simulink model "Galvo_sys_v14"  (R2013a)
settings: Solver=ode45  StartTime=0.0  StopTime=10e-3  MaxStep=1e-4  RelTol=1e-3
InitFcn:
  | Kp_cc = evalin('base','Kp_cc');
StartFcn:
  | Kp_cc = evalin('base','Kp_cc')
model workspace (MATLAB code in the model file):
  | Kp_cc = evalin('base','Kp_cc');
libraries: simulink x2
settings Model: Kp_cc=1  Creator=mainster  LastModifiedBy=mainster
settings DataIOCC: SaveFormat=StructureWithTime

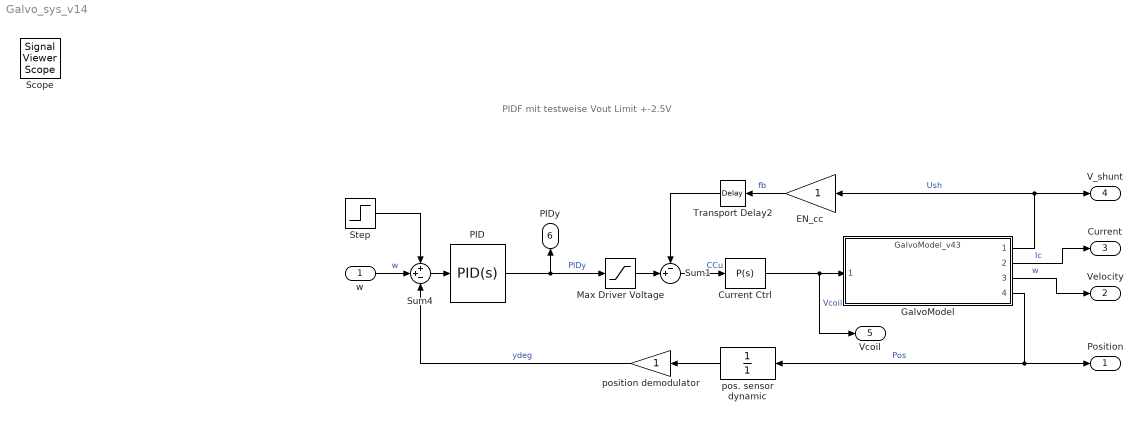
== system Galvo_sys_v14 ==
  note: PIDF mit testweise Vout Limit +-2.5V
  w : Inport
  Current Ctrl : simulink/Continuous/PID Controller  Controller=P  TimeDomain=Continuous-time  SampleTime=1  IntegratorMethod=Forward Euler  FilterMethod=Forward Euler  Form=Parallel  P=Kp_cc  I=1  D=0  N=100  InitialConditionSource=internal  InitialConditionForIntegrator=0  InitialConditionForFilter=0  ExternalReset=none  LimitOutput=off  UpperSaturationLimit=25  LowerSaturationLimit=-25  LinearizeAsGain=on  AntiWindupMode=none  Kb=1  TrackingMode=off  Kt=1  PParamMin=[]  PParamMax=[]  IParamMin=[]  IParamMax=[]  DParamMin=[]  DParamMax=[]  NParamMin=[]  NParamMax=[]  KbParamMin=[]  KbParamMax=[]  KtParamMin=[]  KtParamMax=[]  POutMin=[]  POutMax=[]  IOutMin=[]  IOutMax=[]  DOutMin=[]  DOutMax=[]  NOutMin=[]  NOutMax=[]  KbOutMin=[]  KbOutMax=[]  KtOutMin=[]  KtOutMax=[]  IntegratorOutMin=[]  IntegratorOutMax=[]  FilterOutMin=[]  FilterOutMax=[]  SumOutMin=[]  SumOutMax=[]  SumI1OutMin=[]  SumI1OutMax=[]  SumI2OutMin=[]  SumI2OutMax=[]  SumI3OutMin=[]  SumI3OutMax=[]  SumDOutMin=[]  SumDOutMax=[]  SaturationOutMin=[]  SaturationOutMax=[]  IntegratorContinuousStateAttributes=''  IntegratorStateMustResolveToSignalObject=off  IntegratorRTWStateStorageClass=Auto  FilterContinuousStateAttributes=''  FilterStateMustResolveToSignalObject=off  FilterRTWStateStorageClass=Auto
      settings: AttributesFormatString=Kp_cc=%<P>
  EN_cc : Gain
  GalvoModel : ModelReference  ModelNameDialog=GalvoModel_v43.slx  SimulationMode=Normal  Variant=on  OverrideUsingVariant=GalvoModel_v43  ModelReferenceVersion=1.44  CopyOfModelName=GalvoModel_v43.slx  DefaultDataLogging=on
      mask Display:
      | str=sprintf('%s',get(gcbh,'ModelName'));
      | port_label('input', 1, 'VCoil','texmode','on')
      | color('blue');
      | port_label('output', 1, 'VShunt','texmode','on')
      | color('black');
      | port_label('output', 2, 'Current')
      | port_label('output', 3, 'Velocity')
      | port_label('output', 4, 'Position')
      | %text(.05,.98,['{\fontsize{12}\it\bf' strrep(str,'_',' ') '}'],'horizontalAlignment','left','verticalAlignment','top','texmode','on')
      | text(.015,.98,['{\fontsize{12}\it\bf' strrep(str,'_','\_') '}'],'horizontalAlignment','left','verticalAlignment','top','texmode','on')
  Max Driver Voltage : Saturate  UpperLimit=25  LowerLimit=-25
      settings: AttributesFormatString=VoutMax=+-%<UpperLimit>
  PID : simulink/Continuous/PID Controller  Controller=PID  TimeDomain=Continuous-time  SampleTime=1  IntegratorMethod=Forward Euler  FilterMethod=Forward Euler  Form=Ideal  P=20.0018887757557  I=14.8861285974265  D=0.000703576960586727  N=6270.62036131283  InitialConditionSource=internal  InitialConditionForIntegrator=0  InitialConditionForFilter=0  ExternalReset=none  IgnoreLimit=on  LimitOutput=on  UpperSaturationLimit=25  LowerSaturationLimit=-25  LinearizeAsGain=off  AntiWindupMode=clamping  Kb=6  TrackingMode=off  Kt=0  PParamMin=[]  PParamMax=[]  IParamMin=[]  IParamMax=[]  DParamMin=[]  DParamMax=[]  NParamMin=[]  NParamMax=[]  KbParamMin=[]  KbParamMax=[]  KtParamMin=[]  KtParamMax=[]  POutMin=[]  POutMax=[]  IOutMin=[]  IOutMax=[]  DOutMin=[]  DOutMax=[]  NOutMin=[]  NOutMax=[]  KbOutMin=[]  KbOutMax=[]  KtOutMin=[]  KtOutMax=[]  IntegratorOutMin=[]  IntegratorOutMax=[]  FilterOutMin=[]  FilterOutMax=[]  SumOutMin=[]  SumOutMax=[]  SumI1OutMin=[]  SumI1OutMax=[]  SumI2OutMin=[]  SumI2OutMax=[]  SumI3OutMin=[]  SumI3OutMax=[]  SumDOutMin=[]  SumDOutMax=[]  SaturationOutMin=[]  SaturationOutMax=[]  IntegratorContinuousStateAttributes=''  IntegratorStateMustResolveToSignalObject=off  IntegratorRTWStateStorageClass=Auto  FilterContinuousStateAttributes=''  FilterStateMustResolveToSignalObject=off  FilterRTWStateStorageClass=Auto
      settings: AttributesFormatString=AWM=%<AntiWindupMode>\nD=%<D>\nI=%<I>\nN=%<N>\nP=%<P>\nLimit=+-%<UpperSaturationLimit>
  Step : Step  Time=1e-3  SampleTime=0  ZeroCross=off
      settings: AttributesFormatString=Ampl.: %<After>
  Sum1 : Sum  Inputs=-+|
  Sum4 : Sum  Inputs=++-
  Transport Delay2 : TransportDelay  DelayTime=1e-9
      settings: AttributesFormatString=Delay=%<DelayTime>
  pos. sensor dynamic : TransferFcn  Denominator=[1]
  position demodulator : Gain
  Position : Outport
  Velocity : Outport  Port=2
  Current : Outport  Port=3
  V_shunt : Outport  Port=4
  Vcoil : Outport  Port=5
  PIDy : Outport  Port=6
  Scope : SignalViewerScope  IOType=viewer  NumInputPorts=4  LegendLocations=|  RefreshTime=0.035000
      | 0.78514      0.9169     0.11833    0.028289
      | 0.80649     0.68494       0.129    0.028289
      |       0           0           0           0
      | 0.80472       0.221     0.13968    0.028289
      settings: ShowLegends=on  TimeRange=0.01  YMin=-10~-0.5~-10~-10  YMax=15~1.5~30~30
  wires:
  Sum4/1 -> PID/1
  Step/1 -> Sum4/1
  w/1 -> Sum4/2  "w"
  position demodulator/1 -> Sum4/3  "ydeg"
  GalvoModel/1 -> V_shunt/1, EN_cc/1  "Ush"
  Sum1/1 -> Current Ctrl/1  "CCu"
  PID/1 -> Max Driver Voltage/1, PIDy/1  "PIDy"
  EN_cc/1 -> Transport Delay2/1  "fb"
  Transport Delay2/1 -> Sum1/1
  pos. sensor dynamic/1 -> position demodulator/1
  GalvoModel/4 -> Position/1, pos. sensor dynamic/1  "Pos"
  GalvoModel/2 -> Current/1  "Ic"
  GalvoModel/3 -> Velocity/1  "w"
  Current Ctrl/1 -> GalvoModel/1, Vcoil/1  "Vcoil"
  Max Driver Voltage/1 -> Sum1/2
